simulink model "sim2"  (R2015a)
settings: Solver=ode45  StartTime=0.0  StopTime=10.0  RelTol=1e-3
settings Model: Creator=Martin  LastModifiedBy=Martin

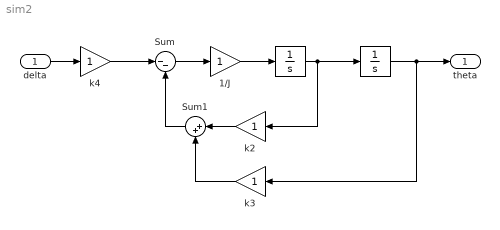
== system sim2 ==
  delta : Inport
  " " : Integrator
  "  " : Integrator
  1/J : Gain
  Sum : Sum  Inputs=|--
  Sum1 : Sum  Inputs=|++
  k2 : Gain
  k3 : Gain
  k4 : Gain
  theta : Outport
  wires:
  delta/1 -> k4/1
  Sum/1 -> 1/J/1
  1/J/1 -> " "/1
  k4/1 -> Sum/1
  " "/1 -> k2/1, "  "/1
  "  "/1 -> k3/1, theta/1
  k2/1 -> Sum1/1
  k3/1 -> Sum1/2
  Sum1/1 -> Sum/2
